simulink model "Ashuganj_South_Main_v020"  (R2024a)
settings: Solver=ode23tb  StartTime=0.0  StopTime=0.1  RelTol=1e-4
undefined symbols (not defined in the file): D1, Delta
libraries: spsThreePhaseTransformerTwoWindingsLib x3, spsThreePhaseParallelRLCLoadLib x3, spsThreePhaseBreakerLib x2, spsThreePhaseSourceLib x2, spsThreePhaseSeriesRLCBranchLib x1, spspowerguiLib x1
settings Model: Creator=Sindid  LastModifiedBy=Sindid
settings DataIOCC: SaveOutput=off  SaveTime=off

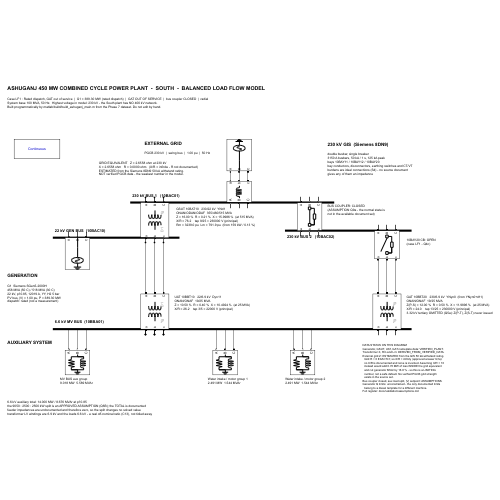
[thumbnail: Simulink's stored preview of the top-level diagram]
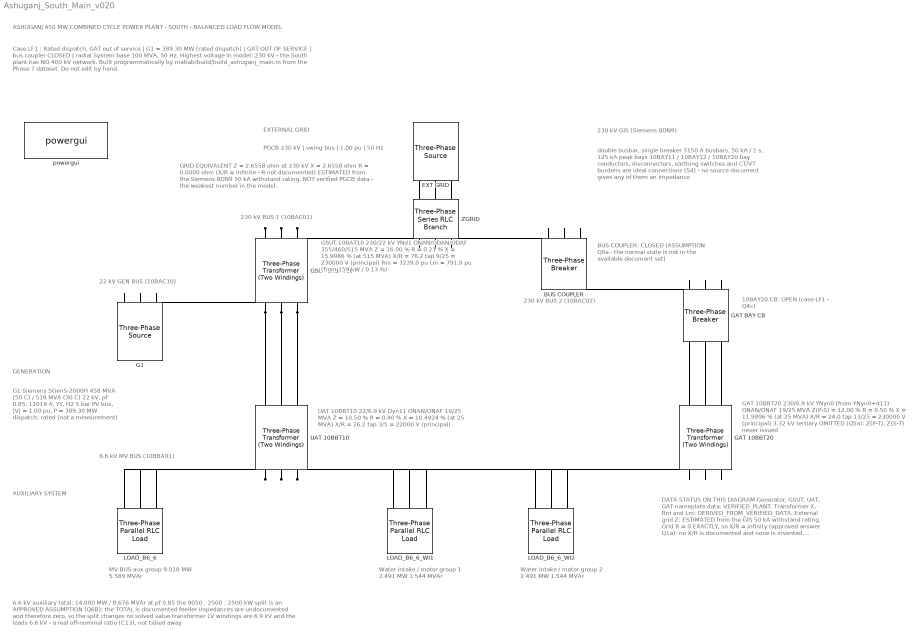
== system Ashuganj_South_Main_v020 ==
  note: EXTERNAL GRID
  note: PGCB 230 kV | swing bus | 1.00 pu | 50 Hz
  note: GRID EQUIVALENT   Z = 2.6558 ohm at 230 kV
      | X = 2.6558 ohm   R = 0.0000 ohm   (X/R = infinite - R not documented)
      | ESTIMATED from the Siemens 8DN9 50 kA withstand rating.
      | NOT verified PGCB data - the weakest number in the model.
  note: GSUT 10BAT10   230/22 kV  YNd1
      | ONAN/ODAN/ODAF  355/460/515 MVA
      | Z = 16.00 %  R = 0.21 %  X = 15.9986 %  (at 515 MVA)
      | X/R = 76.2    tap 9/25 = 230000 V (principal)
      | Rm = 3239.0 pu  Lm = 791.9 pu  (from 159 kW / 0.13 %)
  note: 230 kV GIS (Siemens 8DN9)
  note: double busbar, single breaker
      | 3150 A busbars, 50 kA / 1 s, 125 kA peak
      | bays 10BAY11 / 10BAY12 / 10BAY20
      | bay conductors, disconnectors, earthing switches and CT/VT
      | burdens are ideal connections (S4) - no source document
      | gives any of them an impedance
  note: BUS COUPLER: CLOSED
      | (ASSUMPTION Q9a - the normal state is
      | not in the available document set)
  note: 10BAY20 CB: OPEN
      | (case LF1 - Q4c)
  note: GENERATION
  note: G1  Siemens SGen5-2000H
      | 458 MVA (50 C) / 518 MVA (30 C)
      | 22 kV, pf 0.85, 12019 A, YY, H2 5 bar
      | PV bus, |V| = 1.00 pu, P = 389.30 MW
      | dispatch: rated (not a measurement)
  note: MV BUS aux group
      | 9.018 MW  5.589 MVAr
  note: Water intake / motor group 1
      | 2.491 MW  1.544 MVAr
  note: Water intake / motor group 2
      | 2.491 MW  1.544 MVAr
  note: AUXILIARY SYSTEM
  note: UAT 10BBT10   22/6.9 kV  Dyn11
      | ONAN/ONAF  19/25 MVA
      | Z = 10.50 %  R = 0.40 %  X = 10.4924 %  (at 25 MVA)
      | X/R = 26.2    tap 3/5 = 22000 V (principal)
  note: GAT 10BBT20   230/6.9 kV  YNyn0  (from YNyn0+d11)
      | ONAN/ONAF  19/25 MVA
      | Z(P-S) = 12.00 %  R = 0.50 %  X = 11.9896 %  (at 25 MVA)
      | X/R = 24.0    tap 13/25 = 230000 V (principal)
      | 3.32 kV tertiary OMITTED (Q5a): Z(P-T), Z(S-T) never issued
  note: 6.6 kV auxiliary total: 14.000 MW / 8.676 MVAr at pf 0.85
      | the 9050 : 2500 : 2500 kW split is an APPROVED ASSUMPTION (Q6B); the TOTAL is documented
      | feeder impedances are undocumented and therefore zero, so the split changes no solved value
      | transformer LV windings are 6.9 kV and the loads 6.6 kV - a real off-nominal ratio (C13), not tidied away
  note: 230 kV BUS 1 (10BAC01)
  note: 230 kV BUS 2 (10BAC02)
  note: 22 kV GEN BUS (10BAC10)
  note: 6.6 kV MV BUS (10BBA01)
  note: ASHUGANJ 450 MW COMBINED CYCLE POWER PLANT - SOUTH - BALANCED LOAD FLOW MODEL
  note: Case LF1 : Rated dispatch, GAT out of service  |  G1 = 389.30 MW (rated dispatch)  |  GAT OUT OF SERVICE  |  bus coupler CLOSED  |  radial
      | System base 100 MVA, 50 Hz.  Highest voltage in model: 230 kV - the South plant has NO 400 kV network.
      | Built programmatically by matlab/build/build_ashuganj_main.m from the Phase 7 dataset. Do not edit by hand.
  note: DATA STATUS ON THIS DIAGRAM
      | Generator, GSUT, UAT, GAT nameplate data: VERIFIED_PLANT.
      | Transformer X, Rm and Lm: DERIVED_FROM_VERIFIED_DATA.
      | External grid Z: ESTIMATED from the GIS 50 kA withstand rating.
      |   Grid R = 0 EXACTLY, so X/R = infinity (approved answer Q1a):
      |   no X/R is documented and none is invented. Assuming X/R = 10
      |   instead would add 0.70 MW of loss INSIDE the grid equivalent
      |   and cut generator MVAr by 16.8 % - so this is a LIMITING
      |   number, not a safe default. No verified PGCB grid strength
      |   exists in the source set.
      | Bus coupler closed, aux load split, |V| setpoint: ASSUMPTIONS.
      | Generator Q limits: unconstrained - the only documented limits
      |   belong to a diesel template for a different machine.
      | Full register: docs/validation/assumptions.md
  BUS COUPLER : spsThreePhaseBreakerLib/Three-Phase Breaker  InitialState=closed  SwitchA=on  SwitchB=on  SwitchC=on  SwitchTimes=[1e6]  External=off  BreakerResistance=0.01  SnubberResistance=1e6  SnubberCapacitance=inf  Measurements=None
  EXT GRID : spsThreePhaseSourceLib/Three-Phase Source  InternalConnection=Yg  VoltagePhases=off  Voltage=230000  PhaseAngle=0  Voltage_phases=[25e3 25e3 25e3]/sqrt(3)  PhaseAngles_phases=[0 -120 +120]  Frequency=50  NonIdealSource=off  SpecifyImpedance=off  Resistance=0.8929  Inductance=16.58e-3  ShortCircuitLevel=100e6  BaseVoltage=230000  XRratio=7  BusType=swing  Pref=10e3  Qref=0  Prefabc=[10e3, 10e3, 10e3]  Qrefabc=[0, 0, 0]  Qmin=-inf  Qmax=inf
  G1 : spsThreePhaseSourceLib/Three-Phase Source  InternalConnection=Yg  VoltagePhases=off  Voltage=22000  PhaseAngle=0  Voltage_phases=[25e3 25e3 25e3]/sqrt(3)  PhaseAngles_phases=[0 -120 +120]  Frequency=50  NonIdealSource=off  SpecifyImpedance=off  Resistance=0.8929  Inductance=16.58e-3  ShortCircuitLevel=100e6  BaseVoltage=22000  XRratio=7  BusType=PV  Pref=389300000  Qref=0  Prefabc=[10e3, 10e3, 10e3]  Qrefabc=[0, 0, 0]  Qmin=-inf  Qmax=inf
  GAT 10BBT20 : spsThreePhaseTransformerTwoWindingsLib/Three-Phase Transformer (Two Windings)  Winding1Connection=Yg  Winding2Connection=Yg  CoreType=Three single-phase transformers  SetSaturation=off  Hysteresis=off  DataFile='hysteresis'  SetInitialFlux=off  Measurements=None  UNITS=pu  NominalPower=[ 25000000 , 50 ]  Winding1=[ 230000 , 0.0025 , 0.0599478940414 ]  Winding2=[ 6900 , 0.0025 , 0.0599478940414 ]  Rm=1086.956522  Lm=350.2073842  L0=0.108  Saturation=[ 0,0 ; 0.0024,1.2 ; 1.0,1.52 ]  InitialFluxes=[ 0.8 , -0.8 , 0.7 ]  BreakLoop=off  DiscreteSolver=Trapezoidal iterative  DataType=off  TransfoNumber=1
  GAT BAY CB : spsThreePhaseBreakerLib/Three-Phase Breaker  InitialState=open  SwitchA=on  SwitchB=on  SwitchC=on  SwitchTimes=[1e6]  External=off  BreakerResistance=0.01  SnubberResistance=1e6  SnubberCapacitance=inf  Measurements=None
  GSUT 10BAT10 : spsThreePhaseTransformerTwoWindingsLib/Three-Phase Transformer (Two Windings)  Winding1Connection=Yg  Winding2Connection=Delta (D1)  CoreType=Three single-phase transformers  SetSaturation=off  Hysteresis=off  DataFile='hysteresis'  SetInitialFlux=off  Measurements=None  UNITS=pu  NominalPower=[ 515000000 , 50 ]  Winding1=[ 230000 , 0.00105 , 0.0799931090782 ]  Winding2=[ 22000 , 0.00105 , 0.0799931090782 ]  Rm=3238.993711  Lm=791.8867922  L0=0.158  Saturation=[ 0,0 ; 0.0024,1.2 ; 1.0,1.52 ]  InitialFluxes=[ 0.8 , -0.8 , 0.7 ]  BreakLoop=off  DiscreteSolver=Trapezoidal iterative  DataType=off  TransfoNumber=1
  LOAD_B6_6 : spsThreePhaseParallelRLCLoadLib/Three-Phase Parallel RLC Load  LConnTagsString=A|B|C  Configuration=Y (grounded)  NominalVoltage=6600  Vabc=[1e3 1e3 1e3]  Vabcp=[1e3 1e3 1e3]  NominalFrequency=50  UnbalancedPower=off  ActivePower=9017793.594  InductivePower=5588726.525  CapacitivePower=0  Pabc=[10e3 9e3 11e3]  QLabc=[100 90 110]  QCabc=[100 90 110]  Pabcp=[10e3 9e3 11e3]  QLabcp=[100 90 110]  QCabcp=[100 90 110]  Measurements=None  LoadType=constant PQ
  LOAD_B6_6_WI1 : spsThreePhaseParallelRLCLoadLib/Three-Phase Parallel RLC Load  LConnTagsString=A|B|C  Configuration=Y (grounded)  NominalVoltage=6600  Vabc=[1e3 1e3 1e3]  Vabcp=[1e3 1e3 1e3]  NominalFrequency=50  UnbalancedPower=off  ActivePower=2491103.203  InductivePower=1543847.106  CapacitivePower=0  Pabc=[10e3 9e3 11e3]  QLabc=[100 90 110]  QCabc=[100 90 110]  Pabcp=[10e3 9e3 11e3]  QLabcp=[100 90 110]  QCabcp=[100 90 110]  Measurements=None  LoadType=constant PQ
  LOAD_B6_6_WI2 : spsThreePhaseParallelRLCLoadLib/Three-Phase Parallel RLC Load  LConnTagsString=A|B|C  Configuration=Y (grounded)  NominalVoltage=6600  Vabc=[1e3 1e3 1e3]  Vabcp=[1e3 1e3 1e3]  NominalFrequency=50  UnbalancedPower=off  ActivePower=2491103.203  InductivePower=1543847.106  CapacitivePower=0  Pabc=[10e3 9e3 11e3]  QLabc=[100 90 110]  QCabc=[100 90 110]  Pabcp=[10e3 9e3 11e3]  QLabcp=[100 90 110]  QCabcp=[100 90 110]  Measurements=None  LoadType=constant PQ
  UAT 10BBT10 : spsThreePhaseTransformerTwoWindingsLib/Three-Phase Transformer (Two Windings)  Winding1Connection=Delta (D1)  Winding2Connection=Yg  CoreType=Three single-phase transformers  SetSaturation=off  Hysteresis=off  DataFile='hysteresis'  SetInitialFlux=off  Measurements=None  UNITS=pu  NominalPower=[ 25000000 , 50 ]  Winding1=[ 22000 , 0.002 , 0.0524618909305 ]  Winding2=[ 6900 , 0.002 , 0.0524618909305 ]  Rm=1785.714286  Lm=339.2970532  L0=0.093  Saturation=[ 0,0 ; 0.0024,1.2 ; 1.0,1.52 ]  InitialFluxes=[ 0.8 , -0.8 , 0.7 ]  BreakLoop=off  DiscreteSolver=Trapezoidal iterative  DataType=off  TransfoNumber=1
  ZGRID : spsThreePhaseSeriesRLCBranchLib/Three-Phase Series RLC Branch  LConnTagsString=A|B|C  RConnTagsString=A|B|C  BranchType=L  Resistance=1  Inductance=0.0084537097298  Capacitance=1e-6  Measurements=None
  powergui : spspowerguiLib/powergui  Priority=1  SimulationMode=Continuous  SampleTime=50e-6  frequency=50  Iterations=50  frequencyindice=50  Pbase=100000000  ErrMax=1e-4  UnitsV=kV  UnitsW=MW  buscounter=0  FunctionMessages=off  echomessages=off  EnableUseOfTLC=off  CurrentSourceSwitches=off  DisableSnubberDevices=off  DisableRonSwitches=off  DisableVfSwitches=off  DisplayEquations=off  AutomaticDiscreteSolvers=off  SolverType=Tustin/Backward Euler (TBE)  Interpol=off  ExternalGateDelay=off  methode=off  Ts=100  x0status=blocks  SPID=on  SwTol=0  HookPort=off  NonlinearTolerance=1e-4  nMaxIteration=100  ContinueOnMaxIteration=off  RestoreLinks=warning  ResistiveCurrentMeasurement=off  Frange=[0:2:500]  Ylog=off  Xlog=on  ShowGrid=off  save=off  variable=ZData  structure=0  ZoomFFT=off  StartTime=0.0  cycles=1  DisplayStyle=1  fundamental=60  FreqAxis=off  MaxFrequency=1000  frequencyindicesteady=1  RmsSteady=1  display=off
  connections:
  ZGRID/RConn1 -- EXT GRID/RConn1
  ZGRID/RConn2 -- EXT GRID/RConn2
  ZGRID/RConn3 -- EXT GRID/RConn3
  GAT BAY CB/LConn1 -- BUS COUPLER/RConn1
  GAT BAY CB/LConn2 -- BUS COUPLER/RConn2
  GAT BAY CB/LConn3 -- BUS COUPLER/RConn3
  GAT 10BBT20/RConn1 -- LOAD_B6_6/LConn1 -- LOAD_B6_6_WI1/LConn1 -- UAT 10BBT10/RConn1 -- LOAD_B6_6_WI2/LConn1
  GAT 10BBT20/RConn2 -- LOAD_B6_6/LConn2 -- LOAD_B6_6_WI1/LConn2 -- UAT 10BBT10/RConn2 -- LOAD_B6_6_WI2/LConn2
  GAT 10BBT20/RConn3 -- LOAD_B6_6/LConn3 -- LOAD_B6_6_WI1/LConn3 -- UAT 10BBT10/RConn3 -- LOAD_B6_6_WI2/LConn3
  GSUT 10BAT10/LConn1 -- ZGRID/LConn1 -- BUS COUPLER/LConn1
  GSUT 10BAT10/LConn2 -- ZGRID/LConn2 -- BUS COUPLER/LConn2
  GSUT 10BAT10/LConn3 -- ZGRID/LConn3 -- BUS COUPLER/LConn3
  GSUT 10BAT10/RConn1 -- G1/RConn1 -- UAT 10BBT10/LConn1
  GSUT 10BAT10/RConn2 -- G1/RConn2 -- UAT 10BBT10/LConn2
  GSUT 10BAT10/RConn3 -- G1/RConn3 -- UAT 10BBT10/LConn3
  GAT BAY CB/RConn1 -- GAT 10BBT20/LConn1
  GAT BAY CB/RConn2 -- GAT 10BBT20/LConn2
  GAT BAY CB/RConn3 -- GAT 10BBT20/LConn3
